simulink model "sampleModel931_pp"  (R2021a)
settings: Solver=VariableStepAuto  StartTime=0.0  StopTime=10.0  RelTol=1e-3
undefined symbols (not defined in the file or in its folder): DiscIntNeverNeededParam, magnitude, Newton, Raphson
libraries: simulink x35, pid_lib x8
(part 2 of 2)

== system sampleModel931_pp/cfblk33/cfblk10 ==
  cfblk1 : Inport
  cfblk7 : Inport  Port=2
  cfblk8 : Inport  Port=3
  cfblk3 : Delay  ShowEnablePort=on  SampleTime=1
      settings: InputPortMap=u0,e6
  cfblk4 : DiscreteFir  SampleTime=1
  cfblk5 : DiscreteFir  SampleTime=1
  cfblk6 : ComplexToMagnitudeAngle
  cfblk2 : Outport
  cfblk9 : Outport  Port=2
  wires:
  cfblk6/1 -> cfblk4/1
  cfblk6/2 -> cfblk9/1
  cfblk1/1 -> cfblk5/1
  cfblk4/1 -> cfblk2/1
  cfblk5/1 -> cfblk3/1
  cfblk8/1 -> cfblk3/2
  cfblk7/1 -> cfblk6/1

== system sampleModel931_pp/cfblk33/cfblk11 ==
  cfblk1 : Inport
  cfblk9 : Inport  Port=2
  cfblk10 : Delay  SampleTime=1
  cfblk3 : Math  Operator=log  SaturateOnIntegerOverflow=on
  cfblk4 : Gain  Gain=[-315657696.315725]
  cfblk5 : Sqrt  Operator=rSqrt  AlgorithmType=Newton-Raphson  SaturateOnIntegerOverflow=on
  cfblk6 : simulink/Math Operations/MinMax Running Resettable  Function=min  vinit=0.0
  cfblk7 : Constant  Value=[805415356.666475]  SampleTime=1
  cfblk8 : Constant  Value=[673337076.147362]  SampleTime=1
  cfblk2 : Outport
  wires:
  cfblk6/1 -> cfblk5/1
  cfblk8/1 -> cfblk3/1
  cfblk7/1 -> cfblk2/1
  cfblk9/1 -> cfblk4/1
  cfblk1/1 -> cfblk6/2
  cfblk5/1 -> cfblk10/1
  cfblk10/1 -> cfblk6/1

== system sampleModel931_pp/cfblk33/cfblk9 ==
  cfblk1 : Inport
  cfblk5 : Inport  Port=2
  cfblk6 : Inport  Port=3
  cfblk7 : Inport  Port=4
  cfblk3 : Sqrt  SaturateOnIntegerOverflow=on
  cfblk4 : Sin  TimeSource=Use external signal  SampleTime=0
  cfblk2 : Outport
  cfblk8 : Outport  Port=2
  cfblk9 : Outport  Port=3
  wires:
  cfblk3/1 -> cfblk9/1
  cfblk1/1 -> cfblk4/1
  cfblk7/1 -> cfblk2/1
  cfblk4/1 -> cfblk8/1
  cfblk5/1 -> cfblk3/1

== system sampleModel931_pp/cfblk35/cfblk10 ==
  cfblk1 : Inport
  cfblk9 : Inport  Port=2
  cfblk10 : Inport  Port=3
  cfblk3 : Delay  SampleTime=1
  cfblk4 : DiscreteZeroPole  Poles=[0 0.5]  Gain=1
  cfblk5 : Product  Inputs=**
  cfblk6 : Bias  Bias=[110282203.587144]
  cfblk7 : Squeeze
  cfblk8 : Constant  Value=[602031113.544801]  SampleTime=1
  cfblk2 : Outport
  cfblk11 : Outport  Port=2
  wires:
  cfblk6/1 -> cfblk4/1
  cfblk9/1 -> cfblk6/1
  cfblk10/1 -> cfblk7/1
  cfblk4/1 -> cfblk3/1
  cfblk8/1 -> cfblk11/1
  cfblk3/1 -> cfblk5/1
  cfblk7/1 -> cfblk2/1
  cfblk1/1 -> cfblk5/2

== system sampleModel931_pp/cfblk35/cfblk11 ==
  cfblk1 : Inport
  cfblk12 : Inport  Port=2
  cfblk13 : Inport  Port=3
  cfblk10 : Constant  Value=[-237362533.610093]  SampleTime=1
  cfblk11 : Constant  Value=[664289456.451184]  SampleTime=1
  cfblk3 : pid_lib/PID Controller (2DOF)  Controller=PID  Form=Parallel  TimeDomain=Discrete-time  UseExternalTs=off  SampleTime=1  IntegratorMethod=Forward Euler  FilterMethod=Forward Euler  ControllerParametersSource=internal  P=1  I=1  D=0  UseFilter=on  N=100  b=1  c=1  TunerSelectOption=Transfer Function Based (PID Tuner App)  InitialConditionSource=internal  InitialConditionForIntegrator=0  InitialConditionForFilter=0  DifferentiatorICPrevScaledInput=0  ExternalReset=none  TrackingMode=off  Kt=1  LimitOutput=off  SatLimitsSource=internal  UpperSaturationLimit=inf  LowerSaturationLimit=-inf  LinearizeAsGain=off  AntiWindupMode=none  Kb=1  POutMin=[]  POutMax=[]  IOutMin=[]  IOutMax=[]  DOutMin=[]  DOutMax=[]  NOutMin=[]  NOutMax=[]  bOutMin=[]  bOutMax=[]  cOutMin=[]  cOutMax=[]  SumOutMin=[]  SumOutMax=[]  SaturationOutMin=[]  SaturationOutMax=[]  PParamMin=[]  PParamMax=[]  IParamMin=[]  IParamMax=[]  DParamMin=[]  DParamMax=[]  NParamMin=[]  NParamMax=[]  bParamMin=[]  bParamMax=[]  cParamMin=[]  cParamMax=[]  KbParamMin=[]  KbParamMax=[]  KtParamMin=[]  KtParamMax=[]  KbOutMin=[]  KbOutMax=[]  KtOutMin=[]  KtOutMax=[]  IntegratorOutMin=[]  IntegratorOutMax=[]  FilterOutMin=[]  FilterOutMax=[]  SumI1OutMin=[]  SumI1OutMax=[]  SumI2OutMin=[]  SumI2OutMax=[]  SumI3OutMin=[]  SumI3OutMax=[]  SumI4OutMin=[]  SumI4OutMax=[]  SumDOutMin=[]  SumDOutMax=[]  Sum1OutMin=[]  Sum1OutMax=[]  Sum2OutMin=[]  Sum2OutMax=[]  Sum3OutMin=[]  Sum3OutMax=[]  DifferentiatorOutMin=[]  DifferentiatorOutMax=[]  FilterDiffOutCoefMin=[]  FilterDiffOutCoefMax=[]  ReciprocalOutMin=[]  ReciprocalOutMax=[]  SumDenOutMin=[]  SumDenOutMax=[]  SumNumOutMin=[]  SumNumOutMax=[]  DivideOutMin=[]  DivideOutMax=[]  UdiffTsProdOutMin=[]  UdiffTsProdOutMax=[]  NTsProdOutMin=[]  NTsProdOutMax=[]  UintegralTsProdOutMin=[]  UintegralTsProdOutMax=[]  UngainTsProdOutMin=[]  UngainTsProdOutMax=[]  IntegratorContinuousStateAttributes=''  IntegratorStateMustResolveToSignalObject=off  IntegratorRTWStateStorageClass=Auto  FilterContinuousStateAttributes=''  FilterStateMustResolveToSignalObject=off  FilterRTWStateStorageClass=Auto  ParallelPVariant=InternalParameters  IdealPVariant=Disabled  IVariant=InternalParameters  DVariant=InternalParameters  bVariant=InternalParameters  cVariant=InternalParameters  IntegratorVariant=Discrete  SatVariant=Disabled  AWVariant=Passthrough  PCopyVariant=Disabled  TRVariant=Disabled  FdbkBlocksVariant=Forward  IdealPFdbkVariant=Disabled  SatFdbkVariant=Disabled  DerivativeFilterVariant=ForwardEulerFilter  NVariant=InternalParameters  NCopyVariant=Disabled  FilterICVariant=InternalICsFilter  IntegratorICVariant=InternalICs  ExternalResetVariant=Disabled  TRSumVariant=Passthrough  SumFdbkVariant=Disabled  SumVariant=Sum_PID  TsampFilterVariant=InternalTs  TsampNgainVariant=Passthrough  TsampIntegralVariant=Passthrough  ExternalSaturationOutDataTypeStr=Inherit: Same as second input
      settings: SourceProductBaseCode=SL
  cfblk4 : simulink/Math Operations/MinMax Running Resettable  Function=min  vinit=0.0
  cfblk5 : MinMax  Function=max  Inputs=2
  cfblk6 : UnaryMinus
  cfblk7 : Signum
  cfblk8 : Constant  Value=[770642381.045116]  SampleTime=1
  cfblk9 : Constant  Value=[903124380.080474]  SampleTime=1
  cfblk2 : Outport
  wires:
  cfblk6/1 -> cfblk4/1
  cfblk12/1 -> cfblk3/1
  cfblk8/1 -> cfblk2/1
  cfblk13/1 -> cfblk3/2
  cfblk11/1 -> cfblk7/1
  cfblk7/1 -> cfblk4/2
  cfblk10/1 -> cfblk5/1
  cfblk3/1 -> cfblk5/2
  cfblk1/1 -> cfblk6/1

== system sampleModel931_pp/cfblk35/cfblk12 ==
  cfblk1 : Inport
  cfblk8 : Inport  Port=2
  cfblk9 : Inport  Port=3
  cfblk10 : Inport  Port=4
  cfblk11 : Inport  Port=5
  cfblk12 : Delay  SampleTime=1
  cfblk3 : pid_lib/PID Controller (2DOF)  Controller=PID  Form=Parallel  TimeDomain=Discrete-time  UseExternalTs=off  SampleTime=1  IntegratorMethod=Forward Euler  FilterMethod=Forward Euler  ControllerParametersSource=internal  P=1  I=1  D=0  UseFilter=on  N=100  b=1  c=1  TunerSelectOption=Transfer Function Based (PID Tuner App)  InitialConditionSource=internal  InitialConditionForIntegrator=0  InitialConditionForFilter=0  DifferentiatorICPrevScaledInput=0  ExternalReset=none  TrackingMode=off  Kt=1  LimitOutput=off  SatLimitsSource=internal  UpperSaturationLimit=inf  LowerSaturationLimit=-inf  LinearizeAsGain=off  AntiWindupMode=none  Kb=1  POutMin=[]  POutMax=[]  IOutMin=[]  IOutMax=[]  DOutMin=[]  DOutMax=[]  NOutMin=[]  NOutMax=[]  bOutMin=[]  bOutMax=[]  cOutMin=[]  cOutMax=[]  SumOutMin=[]  SumOutMax=[]  SaturationOutMin=[]  SaturationOutMax=[]  PParamMin=[]  PParamMax=[]  IParamMin=[]  IParamMax=[]  DParamMin=[]  DParamMax=[]  NParamMin=[]  NParamMax=[]  bParamMin=[]  bParamMax=[]  cParamMin=[]  cParamMax=[]  KbParamMin=[]  KbParamMax=[]  KtParamMin=[]  KtParamMax=[]  KbOutMin=[]  KbOutMax=[]  KtOutMin=[]  KtOutMax=[]  IntegratorOutMin=[]  IntegratorOutMax=[]  FilterOutMin=[]  FilterOutMax=[]  SumI1OutMin=[]  SumI1OutMax=[]  SumI2OutMin=[]  SumI2OutMax=[]  SumI3OutMin=[]  SumI3OutMax=[]  SumI4OutMin=[]  SumI4OutMax=[]  SumDOutMin=[]  SumDOutMax=[]  Sum1OutMin=[]  Sum1OutMax=[]  Sum2OutMin=[]  Sum2OutMax=[]  Sum3OutMin=[]  Sum3OutMax=[]  DifferentiatorOutMin=[]  DifferentiatorOutMax=[]  FilterDiffOutCoefMin=[]  FilterDiffOutCoefMax=[]  ReciprocalOutMin=[]  ReciprocalOutMax=[]  SumDenOutMin=[]  SumDenOutMax=[]  SumNumOutMin=[]  SumNumOutMax=[]  DivideOutMin=[]  DivideOutMax=[]  UdiffTsProdOutMin=[]  UdiffTsProdOutMax=[]  NTsProdOutMin=[]  NTsProdOutMax=[]  UintegralTsProdOutMin=[]  UintegralTsProdOutMax=[]  UngainTsProdOutMin=[]  UngainTsProdOutMax=[]  IntegratorContinuousStateAttributes=''  IntegratorStateMustResolveToSignalObject=off  IntegratorRTWStateStorageClass=Auto  FilterContinuousStateAttributes=''  FilterStateMustResolveToSignalObject=off  FilterRTWStateStorageClass=Auto  ParallelPVariant=InternalParameters  IdealPVariant=Disabled  IVariant=InternalParameters  DVariant=InternalParameters  bVariant=InternalParameters  cVariant=InternalParameters  IntegratorVariant=Discrete  SatVariant=Disabled  AWVariant=Passthrough  PCopyVariant=Disabled  TRVariant=Disabled  FdbkBlocksVariant=Forward  IdealPFdbkVariant=Disabled  SatFdbkVariant=Disabled  DerivativeFilterVariant=ForwardEulerFilter  NVariant=InternalParameters  NCopyVariant=Disabled  FilterICVariant=InternalICsFilter  IntegratorICVariant=InternalICs  ExternalResetVariant=Disabled  TRSumVariant=Passthrough  SumFdbkVariant=Disabled  SumVariant=Sum_PID  TsampFilterVariant=InternalTs  TsampNgainVariant=Passthrough  TsampIntegralVariant=Passthrough  ExternalSaturationOutDataTypeStr=Inherit: Same as second input
      settings: SourceProductBaseCode=SL
  cfblk4 : Sum  Inputs=+-
  cfblk5 : Rounding
  cfblk6 : Sum  Inputs=+-
  cfblk7 : Rounding
  cfblk2 : Outport
  wires:
  cfblk8/1 -> cfblk2/1
  cfblk3/1 -> cfblk4/1
  cfblk1/1 -> cfblk5/1
  cfblk9/1 -> cfblk7/1
  cfblk4/1 -> cfblk6/1
  cfblk10/1 -> cfblk6/2
  cfblk5/1 -> cfblk3/1
  cfblk11/1 -> cfblk3/2
  cfblk6/1 -> cfblk12/1
  cfblk12/1 -> cfblk4/2

== system sampleModel931_pp/cfblk35/cfblk13 ==
  cfblk1 : Inport
  cfblk10 : Inport  Port=2
  cfblk11 : Inport  Port=3
  cfblk12 : Inport  Port=4
  cfblk15 : Delay  SampleTime=1
  cfblk3 : DiscreteTransferFcn  SampleTime=1
  cfblk4 : simulink/Discrete/Difference  ICPrevInput=0.0  OutMin=[]  OutMax=[]  OutDataTypeStr=Inherit: Inherit via back propagation  OutDataType=fixdt(1, 16)  OutScaling=2^-10  DoSatur=off
  cfblk5 : simulink/Discrete/Transfer Fcn Real Zero  ZeroZ=0.75  ICPrevInput=0.0  DoSatur=off
      settings: SourceProductBaseCode=SL
  cfblk6 : Sum  Inputs=+-
  cfblk7 : Signum
  cfblk8 : Product
  cfblk9 : Polyval  Coefs=[ +2.081618890e-019, -1.441693666e-014, +4.719686976e-010, -8.536869453e-006, +1.621573104e-001, -8.087801117e+001 ]
  cfblk2 : Outport
  cfblk13 : Outport  Port=2
  cfblk14 : Outport  Port=3
  wires:
  cfblk10/1 -> cfblk14/1
  cfblk1/1 -> cfblk9/1
  cfblk7/1 -> cfblk6/1
  cfblk12/1 -> cfblk3/1, cfblk7/1
  cfblk11/1 -> cfblk2/1
  cfblk9/1 -> cfblk4/1
  cfblk8/1 -> cfblk6/2
  cfblk5/1 -> cfblk8/1
  cfblk4/1 -> cfblk13/1
  cfblk3/1 -> cfblk5/1
  cfblk6/1 -> cfblk15/1
  cfblk15/1 -> cfblk8/2

== system sampleModel931_pp/cfblk35/cfblk14 ==
  cfblk1 : Inport
  cfblk6 : Inport  Port=2
  cfblk3 : DiscreteStateSpace
  cfblk4 : Delay  SampleTime=1
  cfblk5 : Assignment  DiagnosticForDimensions=Warning  IndexOptions=Index vector (dialog)  Indices=1  OutputSizes=1
  cfblk8 : Delay  SampleTime=1
  cfblk2 : Outport
  cfblk7 : Outport  Port=2
  wires:
  cfblk1/1 -> cfblk7/1
  cfblk6/1 -> cfblk5/1
  cfblk3/1 -> cfblk2/1, cfblk4/1
  cfblk4/1 -> cfblk5/2
  cfblk5/1 -> cfblk8/1
  cfblk8/1 -> cfblk3/1

== system sampleModel931_pp/cfblk35/cfblk15 ==
  cfblk1 : Inport
  cfblk13 : Inport  Port=2
  cfblk14 : Inport  Port=3
  cfblk10 : Reshape
  cfblk11 : Constant  Value=[750369943.740463]  SampleTime=1
  cfblk12 : Constant  Value=[805217719.859375]  SampleTime=1
  cfblk16 : Delay  SampleTime=1
  cfblk3 : simulink/Discrete/Difference  ICPrevInput=0.0  OutMin=[]  OutMax=[]  OutDataTypeStr=Inherit: Inherit via back propagation  OutDataType=fixdt(1, 16)  OutScaling=2^-10  DoSatur=off
  cfblk4 : Delay  DelayLengthSource=Input port  SampleTime=1
      settings: InputPortMap=u0,p1
  cfblk5 : simulink/Discrete/Difference  ICPrevInput=0.0  OutMin=[]  OutMax=[]  OutDataTypeStr=Inherit: Inherit via back propagation  OutDataType=fixdt(1, 16)  OutScaling=2^-10  DoSatur=off
  cfblk6 : simulink/Discrete/Transfer Fcn Real Zero  ZeroZ=0.75  ICPrevInput=0.0  DoSatur=off
      settings: SourceProductBaseCode=SL
  cfblk7 : simulink/Math Operations/MinMax Running Resettable  Function=min  vinit=0.0
  cfblk8 : Sqrt  SaturateOnIntegerOverflow=on
  cfblk9 : Sqrt  SaturateOnIntegerOverflow=on
  cfblk2 : Outport
  cfblk15 : Outport  Port=2
  wires:
  cfblk7/1 -> cfblk15/1
  cfblk5/1 -> cfblk2/1
  cfblk4/1 -> cfblk9/1
  cfblk12/1 -> cfblk10/1
  cfblk6/1 -> cfblk4/1
  cfblk11/1 -> cfblk6/1
  cfblk14/1 -> cfblk8/1
  cfblk8/1 -> cfblk3/1
  cfblk1/1 -> cfblk7/1
  cfblk3/1 -> cfblk7/2
  cfblk13/1 -> cfblk5/1
  cfblk9/1 -> cfblk16/1
  cfblk16/1 -> cfblk4/2
